simulink subsystem "TorqueVectoringAlgorithm_subsysref"  (R2020a)
settings: Solver=VariableStepAuto  StartTime=0.0  StopTime=10.0  RelTol=1e-3
libraries: TorqueVectoringAlgorithmLib x1
settings Model: Creator=Kiera  LastModifiedBy=Kiera

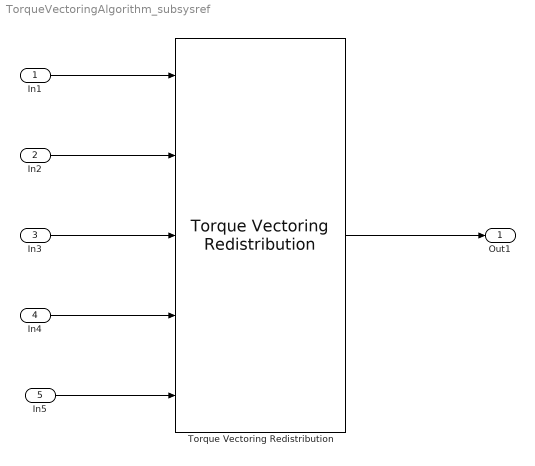
== system TorqueVectoringAlgorithm_subsysref ==
  In1 : Inport
  In2 : Inport  Port=2
  In3 : Inport  Port=3
  In4 : Inport  Port=4
  In5 : Inport  Port=5
  Torque Vectoring Redistribution : TorqueVectoringAlgorithmLib/Torque Vectoring Redistribution  wheel_1=Front  wheel_2=Left
  Out1 : Outport  VectorParamsAs1DForOutWhenUnconnected=off
  wires:
  In2/1 -> Torque Vectoring Redistribution/2
  In5/1 -> Torque Vectoring Redistribution/5
  In4/1 -> Torque Vectoring Redistribution/4
  Torque Vectoring Redistribution/1 -> Out1/1
  In1/1 -> Torque Vectoring Redistribution/1
  In3/1 -> Torque Vectoring Redistribution/3
